simulink model "ques_2_2_simulink"  (R2023b)
settings: Solver=ode1  StartTime=0.0  StopTime=120  FixedStep=0.001  RelTol=1e-3
settings Model: Creator=sarth  LastModifiedBy=sarth

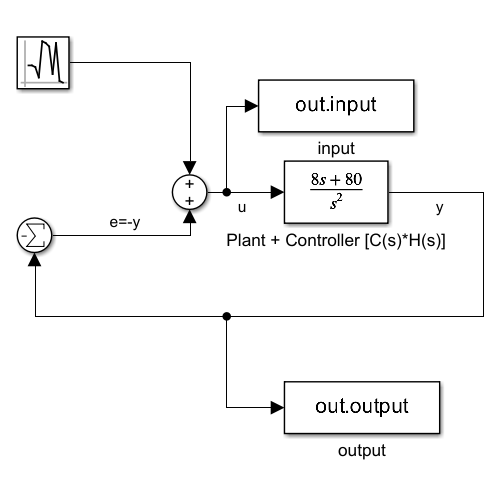
[thumbnail: Simulink's stored preview of the top-level diagram]
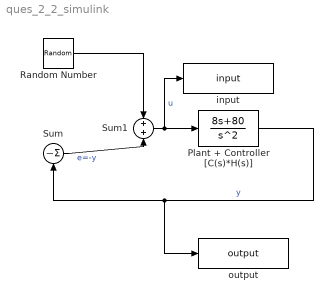
== system ques_2_2_simulink ==
  Plant + Controller [C(s)*H(s)] : TransferFcn  Numerator=[8 80]  Denominator=[1 0 0]
  Random Number : RandomNumber  SampleTime=0.001
  Sum : Sum  Inputs=|-
  Sum1 : Sum
  input : ToWorkspace  VariableName=input  SaveFormat=Timeseries  SampleTime=-1
  output : ToWorkspace  VariableName=output  SaveFormat=Timeseries  SampleTime=-1
  wires:
  Plant + Controller [C(s)*H(s)]/1 -> output/1, Sum/1  "y"
  Sum/1 -> Sum1/2  "e=-y"
  Random Number/1 -> Sum1/1
  Sum1/1 -> input/1, Plant + Controller [C(s)*H(s)]/1  "u"
